simulink model "envelope_detection"  (R2019b)
settings: Solver=VariableStepAuto  StartTime=0.0  StopTime=1  RelTol=1e-3
libraries: simulink x1, dspfdesign x1, dspsrcs4 x1
settings Model: Creator=Siddhartha  LastModifiedBy=Siddhartha

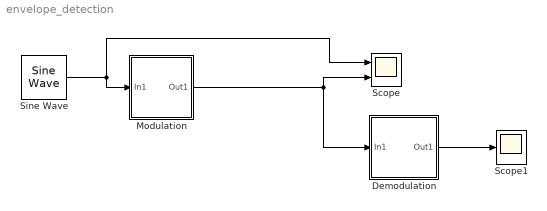
== system envelope_detection ==
  "Demodulation " : Subsystem
  "Modulation " : Subsystem
  Scope : Scope  NumInputPorts=2
  Scope1 : Scope
  Sine Wave : dspsrcs4/Sine Wave  Amplitude=1  Frequency=10  Phase=0  SampleMode=Discrete  OutComplex=Real  CompMethod=Trigonometric fcn  TableSize=Speed  SampleTime=1/15000  SamplesPerFrame=1  ResetState=Restart at time zero  OutputFrames=off  dataType=double  wordLen=16  udDataType=sfix(16)  fracBitsMode=Best precision  numFracBits=15  OutDataTypeStr=double  LastOutDataTypeStr=double
  wires:
  Sine Wave/1 -> "Modulation "/1(In1), Scope/1
  "Modulation "/1(Out1) -> "Demodulation "/1(In1), Scope/2
  "Demodulation "/1(Out1) -> Scope1/1

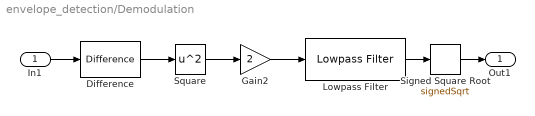
== system envelope_detection/Demodulation  ==
  In1 : Inport
  Difference : simulink/Discrete/Difference  ICPrevInput=0.0  OutMin=[]  OutMax=[]  OutDataType=fixdt(1, 16)  OutScaling=2^-10  DoSatur=off
  Gain2 : Gain  Gain=2
  Lowpass Filter : dspfdesign/Lowpass Filter  FilterType=FIR  DesignForMinimumOrder=on  FilterOrder=50  PassbandFrequency=50  StopbandFrequency=1e2  PassbandRipple=0.1  StopbandAttenuation=80  InheritSampleRate=off  SampleRate=44100  SimulateUsing=Interpreted execution  roundingMode=Floor  coeffsDataTypeStr=fixdt(1,16)
  Signed Square Root : Sqrt  Operator=signedSqrt  SaturateOnIntegerOverflow=on
  Square : Math  Operator=square  SignedPower=off  SaturateOnIntegerOverflow=on
  Out1 : Outport
  wires:
  Gain2/1 -> Lowpass Filter/1
  Square/1 -> Gain2/1
  Lowpass Filter/1 -> Signed Square Root/1
  Signed Square Root/1 -> Out1/1
  Difference/1 -> Square/1
  In1/1 -> Difference/1

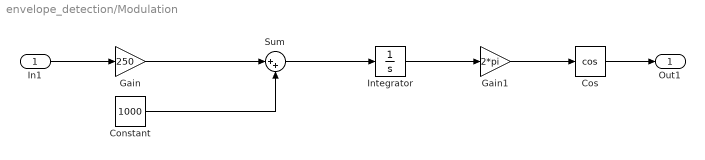
== system envelope_detection/Modulation  ==
  In1 : Inport
  Constant : Constant  Value=1000
  Cos : Trigonometry  Operator=cos
  Gain : Gain  Gain=250
  Gain1 : Gain  Gain=2*pi
  Integrator : Integrator
  Sum : Sum  Inputs=|++
  Out1 : Outport
  wires:
  Gain/1 -> Sum/1
  In1/1 -> Gain/1
  Sum/1 -> Integrator/1
  Constant/1 -> Sum/2
  Cos/1 -> Out1/1
  Gain1/1 -> Cos/1
  Integrator/1 -> Gain1/1
